simulink library "ACT"  (Simulink 10.2)
settings: Solver=VariableStepAuto  StartTime=0.0  StopTime=10.0  RelTol=1e-3
undefined symbols (not defined in the file): ACT_MTR_par
libraries: ACT_MTR x1
settings Model: Creator=dbell44  LastModifiedBy=dbell44

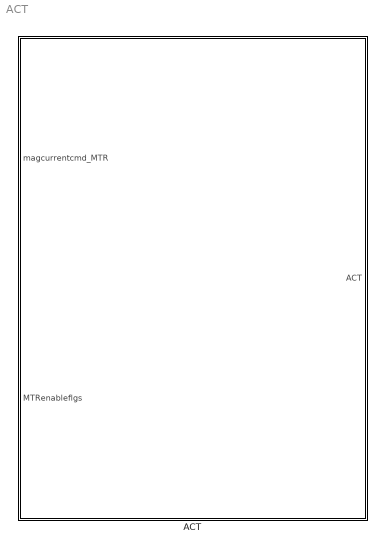
== system ACT ==
  ACT : Subsystem

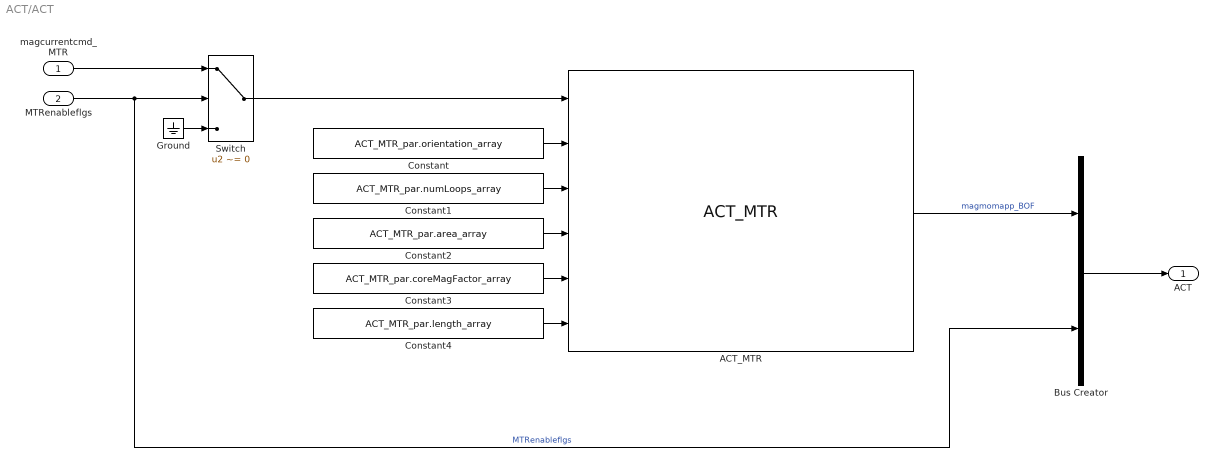
== system ACT/ACT ==
  magcurrentcmd_MTR : Inport
  MTRenableflgs : Inport  Port=2
  ACT_MTR : ACT_MTR/ACT_MTR  SystemSampleTime=-1  VariantActivationTime=update diagram  Latency=0  AutoFrameSizeCalculation=off
  Bus Creator : BusCreator  Inputs=2
  Constant : Constant  Value=ACT_MTR_par.orientation_array
  Constant1 : Constant  Value=ACT_MTR_par.numLoops_array
  Constant2 : Constant  Value=ACT_MTR_par.area_array
  Constant3 : Constant  Value=ACT_MTR_par.coreMagFactor_array
  Constant4 : Constant  Value=ACT_MTR_par.length_array
  Ground : Ground
  Switch : Switch  Criteria=u2 ~= 0
  ACT : Outport
  wires:
  ACT_MTR/1 -> Bus Creator/1  "magmomapp_BOF"
  magcurrentcmd_MTR/1 -> Switch/1
  MTRenableflgs/1 -> Switch/2, Bus Creator/2  "MTRenableflgs"
  Ground/1 -> Switch/3
  Bus Creator/1 -> ACT/1
  Switch/1 -> ACT_MTR/1
  Constant2/1 -> ACT_MTR/4
  Constant1/1 -> ACT_MTR/3
  Constant/1 -> ACT_MTR/2
  Constant3/1 -> ACT_MTR/5
  Constant4/1 -> ACT_MTR/6
